simulink model "test"  (R2018a)
settings: Solver=VariableStepAuto  StartTime=0.0  StopTime=500.0  RelTol=1e-3
values from neighbouring files (symbols this model uses):
  a = normrnd(mu,sigma,2,1)    [main.m]
  w0 = 0.0126    [main.m]
settings Model: Creator=Dantemiwa  LastModifiedBy=Dantemiwa
settings DataIOCC: ReturnWorkspaceOutputs=on
settings SFSimCC: SimUseLocalCustomCode=on
settings RTWCC: RTWUseLocalCustomCode=on

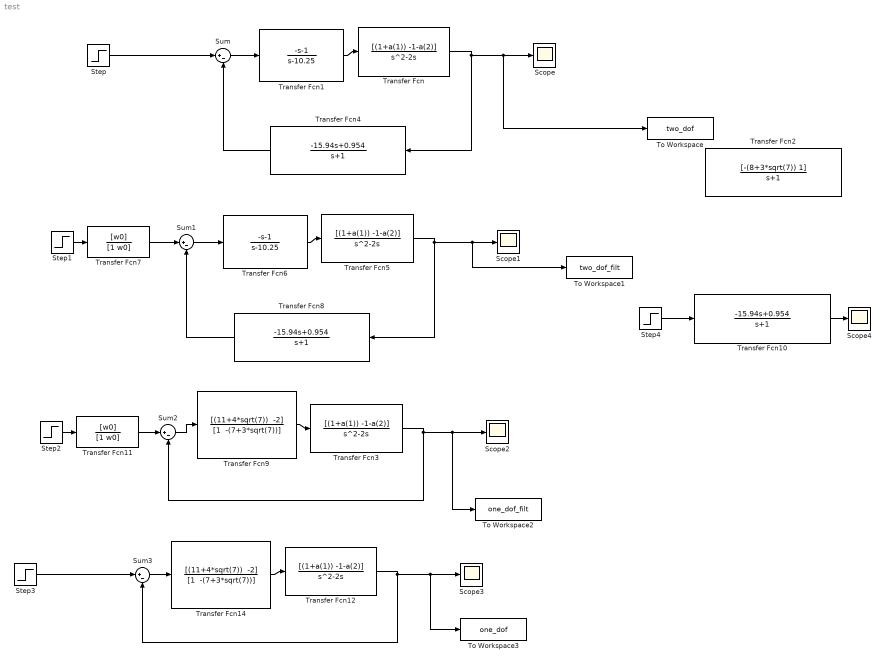
== system test ==
  Scope{,1..4} (5 alike) : Scope
  Step{,1..4} (5 alike) : Step  SampleTime=0
  Sum{,1..3} (4 alike) : Sum  Inputs=|+-
  To Workspace : ToWorkspace  VariableName=two_dof  SampleTime=-1
  To Workspace1 : ToWorkspace  VariableName=two_dof_filt  SampleTime=-1
  To Workspace2 : ToWorkspace  VariableName=one_dof_filt  SampleTime=-1
  To Workspace3 : ToWorkspace  VariableName=one_dof  SampleTime=-1
  Transfer Fcn{,3,5,12} (4 alike) : TransferFcn  Numerator=[(1+a(1)) -1-a(2)]  Denominator=[1 -2 0]
  Transfer Fcn1 : TransferFcn  Numerator=[-1 -1]  Denominator="[1  -10.25]"
  Transfer Fcn10 : TransferFcn  Numerator=[-15.94 0.954]  Denominator=[1 1]
  Transfer Fcn11 : TransferFcn  Numerator=[w0]  Denominator=[1 w0]
  Transfer Fcn14 : TransferFcn  Numerator="[(11+4*sqrt(7))  -2]"  Denominator="[1  -(7+3*sqrt(7))]"
  Transfer Fcn2 : TransferFcn  Numerator=[-(8+3*sqrt(7)) 1]  Denominator=[1 1]
  Transfer Fcn4 : TransferFcn  Numerator=[-15.94 0.954]  Denominator=[1 1]
  Transfer Fcn6 : TransferFcn  Numerator=[-1 -1]  Denominator="[1  -10.25]"
  Transfer Fcn7 : TransferFcn  Numerator=[w0]  Denominator=[1 w0]
  Transfer Fcn8 : TransferFcn  Numerator=[-15.94 0.954]  Denominator=[1 1]
  Transfer Fcn9 : TransferFcn  Numerator="[(11+4*sqrt(7))  -2]"  Denominator="[1  -(7+3*sqrt(7))]"
  wires:
  Transfer Fcn1/1 -> Transfer Fcn/1
  Transfer Fcn/1 -> Transfer Fcn4/1, To Workspace/1, Scope/1
  Transfer Fcn4/1 -> Sum/2
  Sum/1 -> Transfer Fcn1/1
  Step/1 -> Sum/1
  Transfer Fcn5/1 -> Transfer Fcn8/1, To Workspace1/1, Scope1/1
  Sum1/1 -> Transfer Fcn6/1
  Transfer Fcn6/1 -> Transfer Fcn5/1
  Transfer Fcn8/1 -> Sum1/2
  Step1/1 -> Transfer Fcn7/1
  Transfer Fcn7/1 -> Sum1/1
  Transfer Fcn3/1 -> Sum2/2, To Workspace2/1, Scope2/1
  Step2/1 -> Transfer Fcn11/1
  Sum2/1 -> Transfer Fcn9/1
  Transfer Fcn9/1 -> Transfer Fcn3/1
  Transfer Fcn11/1 -> Sum2/1
  Sum3/1 -> Transfer Fcn14/1
  Transfer Fcn14/1 -> Transfer Fcn12/1
  Transfer Fcn12/1 -> Sum3/2, To Workspace3/1, Scope3/1
  Step3/1 -> Sum3/1
  Step4/1 -> Transfer Fcn10/1
  Transfer Fcn10/1 -> Scope4/1
